simulink model "Euler_3DoF"  (R2018b)
settings: Solver=VariableStepAuto  StartTime=0.0  StopTime=20  RelTol=1e-3
model workspace: external: MATLAB File /Users/champion/Documents/MATLAB/Projects/Quadcopter/resources/quadcopter_DataFile.m (data not in the file)
undefined symbols (not defined in the file): sigbuilder_block, smiData, X, Y, Z
libraries: sm_lib x29, nesl_utility x19, simulink x13
(part 2 of 2)

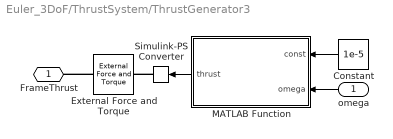
== system Euler_3DoF/ThrustSystem/ThrustGenerator3 ==
  omega : Inport
  Constant : Constant  Value=1e-5
  External Force and Torque : sm_lib/Forces and Torques/External Force and Torque  ForceResolutionFrame=AttachedFrame  EnableForceX=off  EnableForceY=off  EnableForceZ=on  EnableForce=off  TorqueResolutionFrame=AttachedFrame  EnableTorqueX=off  EnableTorqueY=off  EnableTorqueZ=off  EnableTorque=off
  MATLAB Function : MATLAB Function  TreatAsAtomicUnit=on
  Simulink-PS Converter : nesl_utility/Simulink-PS Converter  PhysicalDomain=network_engine_domain  SubClassName=ps_input  LeftPortType=input  RightPortType=output  PseudoPeriodic=off  Frequencies=[]  NoiseDistribution=none  NoiseParameters=[]  Unit=1  AffineConversion=off  FilteringAndDerivatives=provide  SimscapeFilterOrder=1  InputFilterTimeConstant=0.001  UdotUserProvided=0
  FrameThrust : PMIOPort  Side=Right
  wires:
  MATLAB Function/1(thrust) -> Simulink-PS Converter/1
  omega/1 -> MATLAB Function/2(omega)
  Constant/1 -> MATLAB Function/1(const)
  connections:
  External Force and Torque/RConn1 -- FrameThrust/RConn1
  Simulink-PS Converter/RConn1 -- External Force and Torque/LConn1

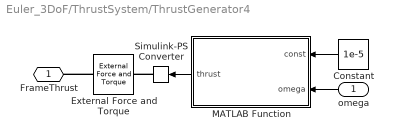
== system Euler_3DoF/ThrustSystem/ThrustGenerator4 ==
  omega : Inport
  Constant : Constant  Value=1e-5
  External Force and Torque : sm_lib/Forces and Torques/External Force and Torque  ForceResolutionFrame=AttachedFrame  EnableForceX=off  EnableForceY=off  EnableForceZ=on  EnableForce=off  TorqueResolutionFrame=AttachedFrame  EnableTorqueX=off  EnableTorqueY=off  EnableTorqueZ=off  EnableTorque=off
  MATLAB Function : MATLAB Function  TreatAsAtomicUnit=on
  Simulink-PS Converter : nesl_utility/Simulink-PS Converter  PhysicalDomain=network_engine_domain  SubClassName=ps_input  LeftPortType=input  RightPortType=output  PseudoPeriodic=off  Frequencies=[]  NoiseDistribution=none  NoiseParameters=[]  Unit=1  AffineConversion=off  FilteringAndDerivatives=provide  SimscapeFilterOrder=1  InputFilterTimeConstant=0.001  UdotUserProvided=0
  FrameThrust : PMIOPort  Side=Right
  wires:
  MATLAB Function/1(thrust) -> Simulink-PS Converter/1
  omega/1 -> MATLAB Function/2(omega)
  Constant/1 -> MATLAB Function/1(const)
  connections:
  External Force and Torque/RConn1 -- FrameThrust/RConn1
  Simulink-PS Converter/RConn1 -- External Force and Torque/LConn1

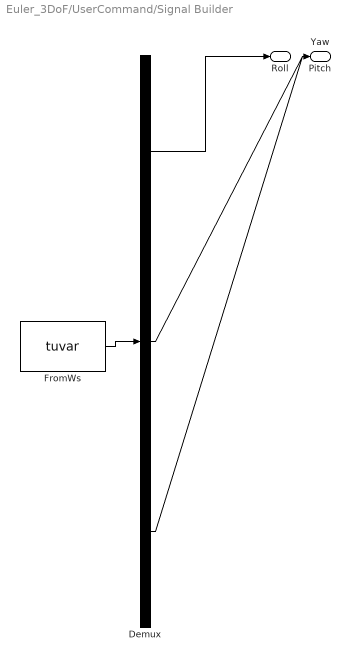
== system Euler_3DoF/UserCommand/Signal Builder ==
  Demux : Demux  Tag=STV Demux  Outputs=3
  FromWs : FromWorkspace  Tag=STV FromWs  VariableName=tuvar  SampleTime=0
      SigBuilderData=|
      | common.afterFinalStr = 'Extrapolate'
      | common.sampleTime = 0
      | dataSet(1).timeRange = [0 10]
      | dataSet(1).name = 'UserTest1'
      | dataSet(2).timeRange = [0 10]
      | dataSet(2).name = 'UserTest2'
      | dataSet(3).timeRange = [0 10]
      | dataSet(3).name = 'UserTest3'
      | dataSet(4).timeRange = [0 10]
      | dataSet(4).name = 'UserTest4'
      | dataSet(5).timeRange = [0 10]
      | dataSet(5).name = 'UserTest5'
      | dataSet(6).timeRange = [0 10]
      | dataSet(6).name = 'StableTest'
      | sbobj.Groups(1).Name = 'UserTest1'
      | sbobj.Groups(1).Signals(1).Name = 'Roll'
      | sbobj.Groups(1).Signals(1).XData = [0 1 1 2 2 10]
      | sbobj.Groups(1).Signals(1).YData = [0 0 0.26 0.26 0 0]
      | sbobj.Groups(1).Signals(2).Name = 'Pitch'
      | sbobj.Groups(1).Signals(2).XData = [0 10]
      | sbobj.Groups(1).Signals(2).YData = [0 0]
      | sbobj.Groups(1).Signals(3).Name = 'Yaw'
      | sbobj.Groups(1).Signals(3).XData = [0 10]
      | sbobj.Groups(1).Signals(3).YData = [0 0]
      | sbobj.Groups(2).Name = 'UserTest2'
      | sbobj.Groups(2).Signals(1).Name = 'Roll'
      | sbobj.Groups(2).Signals(1).XData = [0 10]
      | sbobj.Groups(2).Signals(1).YData = [0 0]
      | sbobj.Groups(2).Signals(2).Name = 'Pitch'
      | sbobj.Groups(2).Signals(2).XData = [0 1 1 2 2 10]
      | sbobj.Groups(2).Signals(2).YData = [0 0 0.26 0.26 0 0]
      | sbobj.Groups(2).Signals(3).Name = 'Yaw'
      | sbobj.Groups(2).Signals(3).XData = [0 10]
      | sbobj.Groups(2).Signals(3).YData = [0 0]
      | sbobj.Groups(3).Name = 'UserTest3'
      | sbobj.Groups(3).Signals(1).Name = 'Roll'
      | sbobj.Groups(3).Signals(1).XData = [0 10]
      | sbobj.Groups(3).Signals(1).YData = [0 0]
      | sbobj.Groups(3).Signals(2).Name = 'Pitch'
      | sbobj.Groups(3).Signals(2).XData = [0 10]
      | sbobj.Groups(3).Signals(2).YData = [0 0]
      | sbobj.Groups(3).Signals(3).Name = 'Yaw'
      | sbobj.Groups(3).Signals(3).XData = [0 2 2 5 5 10]
      | sbobj.Groups(3).Signals(3).YData = [0 0 0.52 0.52 0 0]
      | sbobj.Groups(4).Name = 'UserTest4'
      | sbobj.Groups(4).Signals(1).Name = 'Roll'
      | sbobj.Groups(4).Signals(1).XData = [0 1 1 1.2 1.2 10]
      | sbobj.Groups(4).Signals(1).YData = [0 0 0.26 0.26 0 0]
      | sbobj.Groups(4).Signals(2).Name = 'Pitch'
      | sbobj.Groups(4).Signals(2).XData = [0 4 4 4.2 4.2 10]
      | sbobj.Groups(4).Signals(2).YData = [0 0 0.26 0.26 0 0]
      | sbobj.Groups(4).Signals(3).Name = 'Yaw'
      | sbobj.Groups(4).Signals(3).XData = [0 7 7 8 8 10]
      | sbobj.Groups(4).Signals(3).YData = [0 0 0.26 0.26 0 0]
      | sbobj.Groups(5).Name = 'UserTest5'
      | sbobj.Groups(5).Signals(1).Name = 'Roll'
      | sbobj.Groups(5).Signals(1).XData = [0 1 1 2 2 10]
      | sbobj.Groups(5).Signals(1).YData = [0 0 0.26 0.26 0 0]
      | sbobj.Groups(5).Signals(2).Name = 'Pitch'
      | sbobj.Groups(5).Signals(2).XData = [0 4 4 5 5 10]
      | sbobj.Groups(5).Signals(2).YData = [0 0 0.26 0.26 0 0]
      | sbobj.Groups(5).Signals(3).Name = 'Yaw'
      | sbobj.Groups(5).Signals(3).XData = [0 10]
      | sbobj.Groups(5).Signals(3).YData = [0 0]
      | sbobj.Groups(6).Name = 'StableTest'
      | sbobj.Groups(6).Signals(1).Name = 'Roll'
      | sbobj.Groups(6).Signals(1).XData = [0 10]
      | sbobj.Groups(6).Signals(1).YData = [0 0]
      | sbobj.Groups(6).Signals(2).Name = 'Pitch'
      | sbobj.Groups(6).Signals(2).XData = [0 10]
      | sbobj.Groups(6).Signals(2).YData = [0 0]
      | sbobj.Groups(6).Signals(3).Name = 'Yaw'
      | sbobj.Groups(6).Signals(3).XData = [0 10]
      | sbobj.Groups(6).Signals(3).YData = [0 0]
  Roll : Outport  Tag=STV Outport
  Pitch : Outport  Tag=STV Outport  Port=2
  Yaw : Outport  Tag=STV Outport  Port=3
  wires:
  Demux/1 -> Roll/1
  FromWs/1 -> Demux/1
  Demux/2 -> Pitch/1
  Demux/3 -> Yaw/1

== matlab function Euler_3DoF/ThrustSystem/ThrustGenerator2/MATLAB Function ==
  data: const input; omega input; thrust output
function thrust = CalThrust(const, omega)
    thrust = abs(const * omega^2);

== matlab function Euler_3DoF/ThrustSystem/ThrustGenerator1/MATLAB Function ==
  data: const input; omega input; thrust output
function thrust = CalThrust(const, omega)
    thrust = abs(const * omega^2);

== matlab function Euler_3DoF/ThrustSystem/ThrustGenerator3/MATLAB Function ==
  data: const input; omega input; thrust output
function thrust = CalThrust(const, omega)
    thrust = abs(const * omega^2);

== matlab function Euler_3DoF/ThrustSystem/ThrustGenerator4/MATLAB Function ==
  data: const input; omega input; thrust output
function thrust = CalThrust(const, omega)
    thrust = abs(const * omega^2);
